simulink model "Grid_SensorLayout_SpatialAllignment_Clustering"  (R2018a)
settings: Solver=FixedStepAuto  StartTime=0.0  StopTime=SimulationTime  FixedStep=SamplingTime  RelTol=1e-3
values from neighbouring files (symbols this model uses):
  ValidateGRID = true    [SensorFusion_Script0_main.m]
  ValidateLAYOUT = true    [SensorFusion_Script0_main.m]
  VisualizeCLUSTERING = true    [SensorFusion_Script0_main.m]
undefined symbols (not defined in the file or in its folder): ACTIVATE_CAM, ACTIVATE_RAD, CAM1_detTimeStamp, CAM1_MeasNoise, CAM1_objClassID, CAM1_PX, CAM1_PY, CAM1_VX, CAM1_VY, CAM2_detTimeStamp, CAM2_MeasNoise, CAM2_objClassID, CAM2_PX, CAM2_PY, CAM2_VX, CAM2_VY, CAM3_detTimeStamp, CAM3_MeasNoise, CAM3_objClassID, CAM3_PX, CAM3_PY, CAM3_VX, CAM3_VY, CAM4_detTimeStamp, CAM4_MeasNoise, CAM4_objClassID, CAM4_PX, CAM4_PY, CAM4_VX, CAM4_VY, CAM5_detTimeStamp, CAM5_MeasNoise, CAM5_objClassID, CAM5_PX, CAM5_PY, CAM5_VX, CAM5_VY, CAM6_detTimeStamp, CAM6_MeasNoise, CAM6_objClassID, CAM6_PX, CAM6_PY, CAM6_VX, CAM6_VY, CAM7_detTimeStamp, CAM7_MeasNoise, CAM7_objClassID, CAM7_PX, CAM7_PY, CAM7_VX, CAM7_VY, CAM8_detTimeStamp, CAM8_MeasNoise, CAM8_objClassID, CAM8_PX, CAM8_PY, CAM8_VX, CAM8_VY, CAM_nMeas, CAM_TYPE ... (+171)
libraries: simulink_extras x4
(part 7 of 10)

== system Grid_SensorLayout_SpatialAllignment_Clustering/SENSOR_MEASUREMENTS/RADAR_CAMERA_EGO_SENSOR_INTERFACE/RoadSensors/LineSensor6/Subsystem1 ==
  CameraLineCoeff : Inport
  curv : Inport  Port=2
  curvRate : Inport  Port=3
  curvLen : Inport  Port=4
  alpha : Inport  Port=5
  ValidID : Inport  Port=6
  lateralOffset : Inport  Port=7
  xmin : Inport  Port=8
  xmax : Inport  Port=9
  lineWidth : Inport  Port=10
  TIME_STAMP : Inport  Port=11
  iter : Inport  Port=12
  Assignment : Assignment  DiagnosticForDimensions=Warning  IndexOptions=Index vector (port)  Indices=1  OutputSizes=1
  Bus Creator1 : BusCreator  Inputs=11  OutDataTypeStr=Bus: LineMeasParam  NonVirtualBus=on
  Bus Creator2 : BusCreator  Inputs=11  OutDataTypeStr=Bus: LineMeasParam  NonVirtualBus=on
  Constant1 : Constant  Value=single(10)
  Constant14 : Constant  Value=uint8(6)
  Constant2 : Constant  Value=single(10)
  Constant{35..39,43} (6 alike) : Constant  Value=single(0)
  Constant44 : Constant  Value=single(10)
  Switch : Switch  Criteria=u2 ~= 0
  C1 : Outport
  wires:
  Bus Creator1/1 -> Switch/3
  ValidID/1 -> Bus Creator1/2, Switch/2, Bus Creator2/2  "lineID"
  Bus Creator2/1 -> Switch/1
  CameraLineCoeff/1 -> Assignment/1
  Switch/1 -> Assignment/2
  iter/1 -> Assignment/3
  Assignment/1 -> C1/1
  TIME_STAMP/1 -> Bus Creator2/1  "TimeStamp"
  curv/1 -> Bus Creator2/4  "curvature"
  curvRate/1 -> Bus Creator2/5  "curvatureRate"
  curvLen/1 -> Bus Creator2/6  "curveLength"
  alpha/1 -> Bus Creator2/7  "HeadingAngle"
  lateralOffset/1 -> Bus Creator2/8  "LateralOffset"
  lineWidth/1 -> Bus Creator2/11  "LineMarkWidth"
  xmax/1 -> Bus Creator2/10  "validMinLongCoordLine"
  xmin/1 -> Bus Creator2/9  "validMaxLongCoordLine"
  Constant35/1 -> Bus Creator1/1  "TimeStamp"
  Constant14/1 -> Bus Creator2/3, Bus Creator1/3  "cameraID"
  Constant36/1 -> Bus Creator1/4  "curvature"
  Constant37/1 -> Bus Creator1/5  "curvatureRate"
  Constant38/1 -> Bus Creator1/6  "curveLength"
  Constant39/1 -> Bus Creator1/7  "HeadingAngle"
  Constant43/1 -> Bus Creator1/8  "LateralOffset"
  Constant44/1 -> Bus Creator1/9  "validMaxLongCoordLine"
  Constant1/1 -> Bus Creator1/10  "validMinLongCoordLine"
  Constant2/1 -> Bus Creator1/11  "LineMarkWidth"

== system Grid_SensorLayout_SpatialAllignment_Clustering/SENSOR_MEASUREMENTS/RADAR_CAMERA_EGO_SENSOR_INTERFACE/RoadSensors/LineSensor7/ExtractMeasParam1 ==
  idx : Inport
  time : Inport  Port=2
  Constant : Constant  Value=LINE_CURVATURE_CAM7
  Constant1 : Constant  Value=LINE_CURVDERIVATIVE_CAM7
  Constant2 : Constant  Value=LINE_CURVELENGTH_CAM7
  Constant3 : Constant  Value=LINE_HEADINGANGLE_CAM7
  Constant4 : Constant  Value=LINE_LATERALOFFSET_CAM7
  Constant5 : Constant  Value=LINE_XMIN_CAM7
  Constant6 : Constant  Value=LINE_detTimeStamp_CAM7
  Constant7 : Constant  Value=LINE_XMAX_CAM7
  Constant8 : Constant  Value=LINE_WIDTH_CAM7
  CurvLength : Selector  NumberOfDimensions=2  InputPortWidth=3  IndexOptions=Index vector (port),Index vector (port)  Indices=[1 3],1  OutputSizes=1,1
  Curvature : Selector  NumberOfDimensions=2  InputPortWidth=3  IndexOptions=Index vector (port),Index vector (port)  Indices=[1 3],1  OutputSizes=1,1
  CurvatureRate : Selector  NumberOfDimensions=2  InputPortWidth=3  IndexOptions=Index vector (port),Index vector (port)  Indices=[1 3],1  OutputSizes=1,1
  HeadingAngle : Selector  NumberOfDimensions=2  InputPortWidth=3  IndexOptions=Index vector (port),Index vector (port)  Indices=[1 3],1  OutputSizes=1,1
  LateralOffset : Selector  NumberOfDimensions=2  InputPortWidth=3  IndexOptions=Index vector (port),Index vector (port)  Indices=[1 3],1  OutputSizes=1,1
  lineWidth : Selector  NumberOfDimensions=2  InputPortWidth=3  IndexOptions=Index vector (port),Index vector (port)  Indices=[1 3],1  OutputSizes=1,1
  minValidX : Selector  NumberOfDimensions=2  InputPortWidth=3  IndexOptions=Index vector (port),Index vector (port)  Indices=[1 3],1  OutputSizes=1,1
  minValidY : Selector  NumberOfDimensions=2  InputPortWidth=3  IndexOptions=Index vector (port),Index vector (port)  Indices=[1 3],1  OutputSizes=1,1
  timeStamp : Selector  NumberOfDimensions=2  InputPortWidth=3  IndexOptions=Select all,Index vector (port)  Indices=[1 3],1  OutputSizes=1,1
  curvature : Outport
  curvRate : Outport  Port=2
  curvLength : Outport  Port=3
  headingAngle : Outport  Port=4
  lateralOffset : Outport  Port=5
  xmin : Outport  Port=6
  xmax : Outport  Port=7
  lineMarkWidth : Outport  Port=8
  measCaptureTime : Outport  Port=9
  wires:
  Constant3/1 -> HeadingAngle/1
  Constant2/1 -> CurvLength/1
  HeadingAngle/1 -> headingAngle/1
  Constant/1 -> Curvature/1
  Constant1/1 -> CurvatureRate/1
  CurvLength/1 -> curvLength/1
  Curvature/1 -> curvature/1
  CurvatureRate/1 -> curvRate/1
  Constant4/1 -> LateralOffset/1
  Constant5/1 -> minValidX/1
  Constant6/1 -> timeStamp/1
  timeStamp/1 -> measCaptureTime/1
  minValidX/1 -> xmin/1
  LateralOffset/1 -> lateralOffset/1
  minValidY/1 -> xmax/1
  Constant7/1 -> minValidY/1
  lineWidth/1 -> lineMarkWidth/1
  time/1 -> minValidX/2, minValidY/2, lineWidth/2, timeStamp/2, LateralOffset/2, HeadingAngle/2, CurvLength/2, CurvatureRate/2, Curvature/2
  idx/1 -> minValidX/3, lineWidth/3, minValidY/3, LateralOffset/3, HeadingAngle/3, CurvLength/3, CurvatureRate/3, Curvature/3
  Constant8/1 -> lineWidth/1

== system Grid_SensorLayout_SpatialAllignment_Clustering/SENSOR_MEASUREMENTS/RADAR_CAMERA_EGO_SENSOR_INTERFACE/RoadSensors/LineSensor7/IsValid2 ==
  LineID : Inport
  curvature : Inport  Port=2
  curvatureRate : Inport  Port=3
  curvLength : Inport  Port=4
  HeadingAngle : Inport  Port=5
  Abs{,1..3} (4 alike) : Abs
  Add : Sum  Inputs=++++
  Constant : Constant  Value=uint16(0)
  Data Type Conversion : DataTypeConversion  OutDataTypeStr=uint16
  Switch : Switch  Threshold=0.000001
  validID : Outport
  wires:
  Add/1 -> Switch/2
  Abs2/1 -> Add/3
  Constant/1 -> Switch/3
  Abs/1 -> Add/1
  curvature/1 -> Abs/1
  Abs3/1 -> Add/4
  Abs1/1 -> Add/2
  HeadingAngle/1 -> Abs3/1
  curvatureRate/1 -> Abs1/1
  curvLength/1 -> Abs2/1
  LineID/1 -> Data Type Conversion/1
  Switch/1 -> validID/1
  Data Type Conversion/1 -> Switch/1

== system Grid_SensorLayout_SpatialAllignment_Clustering/SENSOR_MEASUREMENTS/RADAR_CAMERA_EGO_SENSOR_INTERFACE/RoadSensors/LineSensor7/Subsystem1 ==
  CameraLineCoeff : Inport
  curv : Inport  Port=2
  curvRate : Inport  Port=3
  curvLen : Inport  Port=4
  alpha : Inport  Port=5
  ValidID : Inport  Port=6
  lateralOffset : Inport  Port=7
  xmin : Inport  Port=8
  xmax : Inport  Port=9
  lineWidth : Inport  Port=10
  TIME_STAMP : Inport  Port=11
  iter : Inport  Port=12
  Assignment : Assignment  DiagnosticForDimensions=Warning  IndexOptions=Index vector (port)  Indices=1  OutputSizes=1
  Bus Creator1 : BusCreator  Inputs=11  OutDataTypeStr=Bus: LineMeasParam  NonVirtualBus=on
  Bus Creator2 : BusCreator  Inputs=11  OutDataTypeStr=Bus: LineMeasParam  NonVirtualBus=on
  Constant1 : Constant  Value=single(10)
  Constant14 : Constant  Value=uint8(7)
  Constant2 : Constant  Value=single(10)
  Constant{35..39,43} (6 alike) : Constant  Value=single(0)
  Constant44 : Constant  Value=single(10)
  Switch : Switch  Criteria=u2 ~= 0
  C1 : Outport
  wires:
  Bus Creator1/1 -> Switch/3
  ValidID/1 -> Bus Creator1/2, Switch/2, Bus Creator2/2  "lineID"
  Bus Creator2/1 -> Switch/1
  CameraLineCoeff/1 -> Assignment/1
  Switch/1 -> Assignment/2
  iter/1 -> Assignment/3
  Assignment/1 -> C1/1
  TIME_STAMP/1 -> Bus Creator2/1  "TimeStamp"
  curv/1 -> Bus Creator2/4  "curvature"
  curvRate/1 -> Bus Creator2/5  "curvatureRate"
  curvLen/1 -> Bus Creator2/6  "curveLength"
  alpha/1 -> Bus Creator2/7  "HeadingAngle"
  lateralOffset/1 -> Bus Creator2/8  "LateralOffset"
  lineWidth/1 -> Bus Creator2/11  "LineMarkWidth"
  xmax/1 -> Bus Creator2/10  "validMinLongCoordLine"
  xmin/1 -> Bus Creator2/9  "validMaxLongCoordLine"
  Constant35/1 -> Bus Creator1/1  "TimeStamp"
  Constant14/1 -> Bus Creator2/3, Bus Creator1/3  "cameraID"
  Constant36/1 -> Bus Creator1/4  "curvature"
  Constant37/1 -> Bus Creator1/5  "curvatureRate"
  Constant38/1 -> Bus Creator1/6  "curveLength"
  Constant39/1 -> Bus Creator1/7  "HeadingAngle"
  Constant43/1 -> Bus Creator1/8  "LateralOffset"
  Constant44/1 -> Bus Creator1/9  "validMaxLongCoordLine"
  Constant1/1 -> Bus Creator1/10  "validMinLongCoordLine"
  Constant2/1 -> Bus Creator1/11  "LineMarkWidth"

== system Grid_SensorLayout_SpatialAllignment_Clustering/SENSOR_MEASUREMENTS/RADAR_CAMERA_EGO_SENSOR_INTERFACE/RoadSensors/LineSensor8/ExtractMeasParam1 ==
  idx : Inport
  time : Inport  Port=2
  Constant : Constant  Value=LINE_CURVATURE_CAM8
  Constant1 : Constant  Value=LINE_CURVDERIVATIVE_CAM8
  Constant2 : Constant  Value=LINE_CURVELENGTH_CAM8
  Constant3 : Constant  Value=LINE_HEADINGANGLE_CAM8
  Constant4 : Constant  Value=LINE_LATERALOFFSET_CAM8
  Constant5 : Constant  Value=LINE_XMIN_CAM8
  Constant6 : Constant  Value=LINE_detTimeStamp_CAM8
  Constant7 : Constant  Value=LINE_XMAX_CAM8
  Constant8 : Constant  Value=LINE_WIDTH_CAM8
  CurvLength : Selector  NumberOfDimensions=2  InputPortWidth=3  IndexOptions=Index vector (port),Index vector (port)  Indices=[1 3],1  OutputSizes=1,1
  Curvature : Selector  NumberOfDimensions=2  InputPortWidth=3  IndexOptions=Index vector (port),Index vector (port)  Indices=[1 3],1  OutputSizes=1,1
  CurvatureRate : Selector  NumberOfDimensions=2  InputPortWidth=3  IndexOptions=Index vector (port),Index vector (port)  Indices=[1 3],1  OutputSizes=1,1
  HeadingAngle : Selector  NumberOfDimensions=2  InputPortWidth=3  IndexOptions=Index vector (port),Index vector (port)  Indices=[1 3],1  OutputSizes=1,1
  LateralOffset : Selector  NumberOfDimensions=2  InputPortWidth=3  IndexOptions=Index vector (port),Index vector (port)  Indices=[1 3],1  OutputSizes=1,1
  lineWidth : Selector  NumberOfDimensions=2  InputPortWidth=3  IndexOptions=Index vector (port),Index vector (port)  Indices=[1 3],1  OutputSizes=1,1
  minValidX : Selector  NumberOfDimensions=2  InputPortWidth=3  IndexOptions=Index vector (port),Index vector (port)  Indices=[1 3],1  OutputSizes=1,1
  minValidY : Selector  NumberOfDimensions=2  InputPortWidth=3  IndexOptions=Index vector (port),Index vector (port)  Indices=[1 3],1  OutputSizes=1,1
  timeStamp : Selector  NumberOfDimensions=2  InputPortWidth=3  IndexOptions=Select all,Index vector (port)  Indices=[1 3],1  OutputSizes=1,1
  curvature : Outport
  curvRate : Outport  Port=2
  curvLength : Outport  Port=3
  headingAngle : Outport  Port=4
  lateralOffset : Outport  Port=5
  xmin : Outport  Port=6
  xmax : Outport  Port=7
  lineMarkWidth : Outport  Port=8
  measCaptureTime : Outport  Port=9
  wires:
  Constant3/1 -> HeadingAngle/1
  Constant2/1 -> CurvLength/1
  HeadingAngle/1 -> headingAngle/1
  Constant/1 -> Curvature/1
  Constant1/1 -> CurvatureRate/1
  CurvLength/1 -> curvLength/1
  Curvature/1 -> curvature/1
  CurvatureRate/1 -> curvRate/1
  Constant4/1 -> LateralOffset/1
  Constant5/1 -> minValidX/1
  Constant6/1 -> timeStamp/1
  timeStamp/1 -> measCaptureTime/1
  minValidX/1 -> xmin/1
  LateralOffset/1 -> lateralOffset/1
  minValidY/1 -> xmax/1
  Constant7/1 -> minValidY/1
  lineWidth/1 -> lineMarkWidth/1
  time/1 -> minValidX/2, minValidY/2, lineWidth/2, timeStamp/2, LateralOffset/2, HeadingAngle/2, CurvLength/2, CurvatureRate/2, Curvature/2
  idx/1 -> minValidX/3, lineWidth/3, minValidY/3, LateralOffset/3, HeadingAngle/3, CurvLength/3, CurvatureRate/3, Curvature/3
  Constant8/1 -> lineWidth/1

== system Grid_SensorLayout_SpatialAllignment_Clustering/SENSOR_MEASUREMENTS/RADAR_CAMERA_EGO_SENSOR_INTERFACE/RoadSensors/LineSensor8/IsValid2 ==
  LineID : Inport
  curvature : Inport  Port=2
  curvatureRate : Inport  Port=3
  curvLength : Inport  Port=4
  HeadingAngle : Inport  Port=5
  Abs{,1..3} (4 alike) : Abs
  Add : Sum  Inputs=++++
  Constant : Constant  Value=uint16(0)
  Data Type Conversion : DataTypeConversion  OutDataTypeStr=uint16
  Switch : Switch  Threshold=0.000001
  validID : Outport
  wires:
  Add/1 -> Switch/2
  Abs2/1 -> Add/3
  Constant/1 -> Switch/3
  Abs/1 -> Add/1
  curvature/1 -> Abs/1
  Abs3/1 -> Add/4
  Abs1/1 -> Add/2
  HeadingAngle/1 -> Abs3/1
  curvatureRate/1 -> Abs1/1
  curvLength/1 -> Abs2/1
  LineID/1 -> Data Type Conversion/1
  Switch/1 -> validID/1
  Data Type Conversion/1 -> Switch/1

== system Grid_SensorLayout_SpatialAllignment_Clustering/SENSOR_MEASUREMENTS/RADAR_CAMERA_EGO_SENSOR_INTERFACE/RoadSensors/LineSensor8/Subsystem1 ==
  CameraLineCoeff : Inport
  curv : Inport  Port=2
  curvRate : Inport  Port=3
  curvLen : Inport  Port=4
  alpha : Inport  Port=5
  ValidID : Inport  Port=6
  lateralOffset : Inport  Port=7
  xmin : Inport  Port=8
  xmax : Inport  Port=9
  lineWidth : Inport  Port=10
  TIME_STAMP : Inport  Port=11
  iter : Inport  Port=12
  Assignment : Assignment  DiagnosticForDimensions=Warning  IndexOptions=Index vector (port)  Indices=1  OutputSizes=1
  Bus Creator1 : BusCreator  Inputs=11  OutDataTypeStr=Bus: LineMeasParam  NonVirtualBus=on
  Bus Creator2 : BusCreator  Inputs=11  OutDataTypeStr=Bus: LineMeasParam  NonVirtualBus=on
  Constant1 : Constant  Value=single(10)
  Constant14 : Constant  Value=uint8(8)
  Constant2 : Constant  Value=single(10)
  Constant{35..39,43} (6 alike) : Constant  Value=single(0)
  Constant44 : Constant  Value=single(10)
  Switch : Switch  Criteria=u2 ~= 0
  C1 : Outport
  wires:
  Bus Creator1/1 -> Switch/3
  ValidID/1 -> Bus Creator1/2, Switch/2, Bus Creator2/2  "lineID"
  Bus Creator2/1 -> Switch/1
  CameraLineCoeff/1 -> Assignment/1
  Switch/1 -> Assignment/2
  iter/1 -> Assignment/3
  Assignment/1 -> C1/1
  TIME_STAMP/1 -> Bus Creator2/1  "TimeStamp"
  curv/1 -> Bus Creator2/4  "curvature"
  curvRate/1 -> Bus Creator2/5  "curvatureRate"
  curvLen/1 -> Bus Creator2/6  "curveLength"
  alpha/1 -> Bus Creator2/7  "HeadingAngle"
  lateralOffset/1 -> Bus Creator2/8  "LateralOffset"
  lineWidth/1 -> Bus Creator2/11  "LineMarkWidth"
  xmax/1 -> Bus Creator2/10  "validMinLongCoordLine"
  xmin/1 -> Bus Creator2/9  "validMaxLongCoordLine"
  Constant35/1 -> Bus Creator1/1  "TimeStamp"
  Constant14/1 -> Bus Creator2/3, Bus Creator1/3  "cameraID"
  Constant36/1 -> Bus Creator1/4  "curvature"
  Constant37/1 -> Bus Creator1/5  "curvatureRate"
  Constant38/1 -> Bus Creator1/6  "curveLength"
  Constant39/1 -> Bus Creator1/7  "HeadingAngle"
  Constant43/1 -> Bus Creator1/8  "LateralOffset"
  Constant44/1 -> Bus Creator1/9  "validMaxLongCoordLine"
  Constant1/1 -> Bus Creator1/10  "validMinLongCoordLine"
  Constant2/1 -> Bus Creator1/11  "LineMarkWidth"

== system Grid_SensorLayout_SpatialAllignment_Clustering/OBJECT_TRACKER_SENSOR_FUSION/NEAREST_NEIGHBOUR_FOR_CAMERA_MEASUREMENT_GROUPING/NN_MEASUREMENT_GROUPING_WITHIN_EPS/For Iterator Subsystem/NN/PERFORM_NN_CLUSTERING ==
  nMeas : Inport
  measArray : Inport  Port=2
  CLSTR_DATA : Inport  Port=3
  idx_i : Inport  Port=4
  CHECK_CONDITION : Subsystem
  For Iterator : ForIterator  ResetStates=reset  IterationSource=external
  SET_DATA : Subsystem
  CLSTR_DATA_UPD : Outport
  wires:
  nMeas/1 -> For Iterator/1
  idx_i/1 -> CHECK_CONDITION/2(idx_i)
  measArray/1 -> CHECK_CONDITION/1(MEAS)
  For Iterator/1 -> [y_j], CHECK_CONDITION/3(idx_j)
  CHECK_CONDITION/1(isMember) -> SET_DATA/1(isClusterMember)
  SET_DATA/1(CLSTR_DATA_UPD) -> CHECK_CONDITION/5(CLSTR_DATA_PREV), CLSTR_DATA_UPD/1
  CLSTR_DATA/1 -> CHECK_CONDITION/4(CLSTR_DATA_INIT)
  CHECK_CONDITION/2(CLSTR_DATA) -> SET_DATA/2(CLSTR_DATA)
  [y_j] -> SET_DATA/3(idx_j)

== system Grid_SensorLayout_SpatialAllignment_Clustering/OBJECT_TRACKER_SENSOR_FUSION/NEAREST_NEIGHBOUR_FOR_CAMERA_MEASUREMENT_GROUPING/NN_MEASUREMENT_GROUPING_WITHIN_EPS/For Iterator Subsystem/NN/SET_CLUSTER_ID_AND_UPDATE_NUMBER_OF_CLUSTERS ==
  CLUSTERING_DATA : Inport
  CAM_MEAS_CTS : Inport  Port=2
  Add2 : Sum
  Bus Creator : BusCreator  Inputs=7  OutDataTypeStr=Bus: CLUSTER_DATA_STRUCT_SNSR  NonVirtualBus=on
      settings: InheritFromInputs=off
  Bus Selector : BusSelector  OutputSignals=nClusters
  Bus Selector1 : BusSelector  OutputSignals=ValidCumulativeMeasCount
  Bus Selector2 : BusSelector  OutputSignals=ClusterCenter,ClusterCovariance,ClusterSizes,ClusterToMeasAssignment,isMeasVisitedFlag,nClusters,ClusterMember
  Constant3 : Constant  Value=uint16(1)
  Data Type Conversion : DataTypeConversion  OutDataTypeStr=uint16
  Selector : Selector  NumberOfDimensions=2  InputPortWidth=3  IndexOptions=Select all,Index vector (port)  Indices=[1 3],1  OutputSizes=1,1
  Terminator1 : Terminator
  Width : Width
  nRadMeas : Outport
  CLUSTER_DATA : Outport  Port=2
  wires:
  CLUSTERING_DATA/1 -> Bus Selector2/1, Bus Selector/1
  Bus Selector/1 -> Add2/1  "<nClusters>"
  CAM_MEAS_CTS/1 -> Bus Selector1/1
  Add2/1 -> Data Type Conversion/1
  Constant3/1 -> Add2/2
  Data Type Conversion/1 -> [B]
  Bus Selector2/1 -> Bus Creator/1  "<ClusterCenter>"
  Bus Selector2/2 -> Bus Creator/2  "<ClusterCovariance>"
  Bus Selector2/3 -> Bus Creator/3  "<ClusterSizes>"
  Bus Selector2/4 -> Bus Creator/4  "<ClusterToMeasAssignment>"
  Bus Selector2/5 -> Bus Creator/5  "<isMeasVisitedFlag>"
  Bus Selector2/7 -> Bus Creator/7  "<ClusterMember>"
  Bus Selector2/6 -> Terminator1/1  "<nClusters>"
  [B] -> Bus Creator/6  "nClusters"
  Bus Creator/1 -> CLUSTER_DATA/1
  Bus Selector1/1 -> Width/1, Selector/1  "<ValidCumulativeMeasCount>"
  Width/1 -> Selector/2
  Selector/1 -> nRadMeas/1

== system Grid_SensorLayout_SpatialAllignment_Clustering/OBJECT_TRACKER_SENSOR_FUSION/NEAREST_NEIGHBOUR_FOR_CAMERA_MEASUREMENT_GROUPING/NN_MEASUREMENT_GROUPING_WITHIN_EPS/For Iterator Subsystem/NN/Subsystem ==
  CLSTR_DATA : Inport
  Bus Selector : BusSelector  OutputSignals=ClusterSizes,nClusters
  Selector : Selector  NumberOfDimensions=2  InputPortWidth=3  IndexOptions=Select all,Index vector (port)  Indices=[1 3],1  OutputSizes=1,1
  ClstrSize : Outport
  wires:
  Bus Selector/2 -> Selector/2  "<nClusters>"
  Bus Selector/1 -> Selector/1  "<ClusterSizes>"
  CLSTR_DATA/1 -> Bus Selector/1
  Selector/1 -> ClstrSize/1

== system Grid_SensorLayout_SpatialAllignment_Clustering/OBJECT_TRACKER_SENSOR_FUSION/SENSOR_LAYOUT_AND_CHRACTERIZATION/PRE_COMPUTE_SENSOR_FOV_GRID/COMPUTE_CAMERA_SNSR_GRID/ComputeCoverageANDConfidence/Compute_Cell_X_and_Y_index ==
  CellIndex : Inport
  GridID_vec : Inport  Port=2
  GridParam : Inport  Port=3
  SensorExtrinsicParam : Inport  Port=4
  SensorIntrinsicParam : Inport  Port=5
  Compute_Cell_X_Y_Center_Coordinate : Subsystem
  Compute_FOV_Overlap_with_Cell_and_Region_Confidence : Subsystem
  GET_DATA : Subsystem
  Transform_Cell_Coordinate_Vehicle_Frame_To_Sensor_Frame : Subsystem
  RegionConfidence : Outport
  FOVOverlap : Outport  Port=2
  wires:
  GridID_vec/1 -> GET_DATA/1(GridID_vector)
  CellIndex/1 -> GET_DATA/2(index)
  GridParam/1 -> GET_DATA/3(GridParam)
  GET_DATA/1(CellID) -> Compute_Cell_X_Y_Center_Coordinate/1(Cell_id)
  GET_DATA/2(<xRes>) -> Compute_Cell_X_Y_Center_Coordinate/2(xRes)
  GET_DATA/3(<xRear>) -> Compute_Cell_X_Y_Center_Coordinate/3(xRear)
  GET_DATA/4(<nGridCellsLat>) -> Compute_Cell_X_Y_Center_Coordinate/4(Cy)
  GET_DATA/5(<yRes>) -> Compute_Cell_X_Y_Center_Coordinate/5(yRes)
  GET_DATA/6(<yLeft>) -> Compute_Cell_X_Y_Center_Coordinate/6(yLeft)
  SensorExtrinsicParam/1 -> Transform_Cell_Coordinate_Vehicle_Frame_To_Sensor_Frame/3(SensorExtrinsic)
  Compute_Cell_X_Y_Center_Coordinate/1(CellCenterCoordX) -> Transform_Cell_Coordinate_Vehicle_Frame_To_Sensor_Frame/1(Cell_xCoord)
  Compute_Cell_X_Y_Center_Coordinate/2(CellCenterCoordY) -> Transform_Cell_Coordinate_Vehicle_Frame_To_Sensor_Frame/2(Cell_y_Coord)
  Transform_Cell_Coordinate_Vehicle_Frame_To_Sensor_Frame/1(Cell_xSnsrCoord) -> Compute_FOV_Overlap_with_Cell_and_Region_Confidence/1(Cell_xSnsrCoord)
  Transform_Cell_Coordinate_Vehicle_Frame_To_Sensor_Frame/2(Cell_ySnsrCoord) -> Compute_FOV_Overlap_with_Cell_and_Region_Confidence/2(Cell_ySnsrCoord)
  SensorIntrinsicParam/1 -> Compute_FOV_Overlap_with_Cell_and_Region_Confidence/3(SnsrIntrinsic)
  Compute_FOV_Overlap_with_Cell_and_Region_Confidence/1(RegionConfidence) -> RegionConfidence/1
  Compute_FOV_Overlap_with_Cell_and_Region_Confidence/2(FOVOverlap) -> FOVOverlap/1

== system Grid_SensorLayout_SpatialAllignment_Clustering/OBJECT_TRACKER_SENSOR_FUSION/SENSOR_LAYOUT_AND_CHRACTERIZATION/PRE_COMPUTE_SENSOR_FOV_GRID/COMPUTE_CAMERA_SNSR_GRID/ComputeCoverageANDConfidence/SET_DATA ==
  GridIndex : Inport
  RegionConfiArray : Inport  Port=2
  FOVOverlapArray : Inport  Port=3
  SnsrIndex : Inport  Port=4
  confi : Inport  Port=5
  overlap : Inport  Port=6
  Assignment : Assignment  NumberOfDimensions=2  DiagnosticForDimensions=Warning  IndexOptions=Index vector (port),Index vector (port)  Indices=1,1  OutputSizes=1,1
  Assignment1 : Assignment  NumberOfDimensions=2  DiagnosticForDimensions=Warning  IndexOptions=Index vector (port),Index vector (port)  Indices=1,1  OutputSizes=1,1
  RegionConfidence : Outport
  FOVOverlap : Outport  Port=2
  wires:
  SnsrIndex/1 -> Assignment1/3, Assignment/3
  RegionConfiArray/1 -> Assignment/1
  Assignment/1 -> RegionConfidence/1
  GridIndex/1 -> Assignment/4, Assignment1/4
  Assignment1/1 -> FOVOverlap/1
  overlap/1 -> Assignment1/2
  FOVOverlapArray/1 -> Assignment1/1
  confi/1 -> Assignment/2

== system Grid_SensorLayout_SpatialAllignment_Clustering/OBJECT_TRACKER_SENSOR_FUSION/SENSOR_LAYOUT_AND_CHRACTERIZATION/PRE_COMPUTE_SENSOR_FOV_GRID/COMPUTE_RADAR_SNSR_GRID/ComputeCoverageANDConfidence/Compute_Cell_X_and_Y_index ==
  CellIndex : Inport
  GridID_vec : Inport  Port=2
  GridParam : Inport  Port=3
  SensorExtrinsicParam : Inport  Port=4
  SensorIntrinsicParam : Inport  Port=5
  Compute_Cell_X_Y_Center_Coordinate : Subsystem
  Compute_FOV_Overlap_with_Cell_and_Region_Confidence : Subsystem
  GET_DATA : Subsystem
  Transform_Cell_Coordinate_Vehicle_Frame_To_Sensor_Frame : Subsystem
  RegionConfidence : Outport
  FOVOverlap : Outport  Port=2
  wires:
  GridID_vec/1 -> GET_DATA/1(GridID_vector)
  CellIndex/1 -> GET_DATA/2(index)
  GridParam/1 -> GET_DATA/3(GridParam)
  GET_DATA/1(CellID) -> Compute_Cell_X_Y_Center_Coordinate/1(Cell_id)
  GET_DATA/2(<xRes>) -> Compute_Cell_X_Y_Center_Coordinate/2(xRes)
  GET_DATA/3(<xRear>) -> Compute_Cell_X_Y_Center_Coordinate/3(xRear)
  GET_DATA/4(<nGridCellsLat>) -> Compute_Cell_X_Y_Center_Coordinate/4(Cy)
  GET_DATA/5(<yRes>) -> Compute_Cell_X_Y_Center_Coordinate/5(yRes)
  GET_DATA/6(<yLeft>) -> Compute_Cell_X_Y_Center_Coordinate/6(yLeft)
  SensorExtrinsicParam/1 -> Transform_Cell_Coordinate_Vehicle_Frame_To_Sensor_Frame/3(SensorExtrinsic)
  Compute_Cell_X_Y_Center_Coordinate/1(CellCenterCoordX) -> Transform_Cell_Coordinate_Vehicle_Frame_To_Sensor_Frame/1(Cell_xCoord)
  Compute_Cell_X_Y_Center_Coordinate/2(CellCenterCoordY) -> Transform_Cell_Coordinate_Vehicle_Frame_To_Sensor_Frame/2(Cell_y_Coord)
  Transform_Cell_Coordinate_Vehicle_Frame_To_Sensor_Frame/1(Cell_xSnsrCoord) -> Compute_FOV_Overlap_with_Cell_and_Region_Confidence/1(Cell_xSnsrCoord)
  Transform_Cell_Coordinate_Vehicle_Frame_To_Sensor_Frame/2(Cell_ySnsrCoord) -> Compute_FOV_Overlap_with_Cell_and_Region_Confidence/2(Cell_ySnsrCoord)
  SensorIntrinsicParam/1 -> Compute_FOV_Overlap_with_Cell_and_Region_Confidence/3(SnsrIntrinsic)
  Compute_FOV_Overlap_with_Cell_and_Region_Confidence/1(RegionConfidence) -> RegionConfidence/1
  Compute_FOV_Overlap_with_Cell_and_Region_Confidence/2(FOVOverlap) -> FOVOverlap/1

== system Grid_SensorLayout_SpatialAllignment_Clustering/OBJECT_TRACKER_SENSOR_FUSION/SENSOR_LAYOUT_AND_CHRACTERIZATION/PRE_COMPUTE_SENSOR_FOV_GRID/COMPUTE_RADAR_SNSR_GRID/ComputeCoverageANDConfidence/SET_DATA ==
  GridIndex : Inport
  RegionConfiArray : Inport  Port=2
  FOVOverlapArray : Inport  Port=3
  SnsrIndex : Inport  Port=4
  confi : Inport  Port=5
  overlap : Inport  Port=6
  Assignment : Assignment  NumberOfDimensions=2  DiagnosticForDimensions=Warning  IndexOptions=Index vector (port),Index vector (port)  Indices=1,1  OutputSizes=1,1
  Assignment1 : Assignment  NumberOfDimensions=2  DiagnosticForDimensions=Warning  IndexOptions=Index vector (port),Index vector (port)  Indices=1,1  OutputSizes=1,1
  RegionConfidence : Outport
  FOVOverlap : Outport  Port=2
  wires:
  SnsrIndex/1 -> Assignment1/3, Assignment/3
  RegionConfiArray/1 -> Assignment/1
  Assignment/1 -> RegionConfidence/1
  GridIndex/1 -> Assignment/4, Assignment1/4
  Assignment1/1 -> FOVOverlap/1
  overlap/1 -> Assignment1/2
  FOVOverlapArray/1 -> Assignment1/1
  confi/1 -> Assignment/2

== system Grid_SensorLayout_SpatialAllignment_Clustering/OBJECT_TRACKER_SENSOR_FUSION/SENSOR_LAYOUT_AND_CHRACTERIZATION/PRE_COMPUTE_SENSOR_FOV_GRID/CREATE_GRID/For Iterator Subsystem/Compute_Grid_Cell_Cartesian_Coordinate ==
  note: Get_Grid_Limits_Data
  note: Compute_Grid_Cell_x_Coordinate
  note: Compute_Grid_Cell_y_Coordinate
  GridParam : Inport
  x_Index : Inport  Port=2
  y_Index : Inport  Port=3
  Add : Sum
  Add1 : Sum
  Bus Selector : BusSelector  OutputSignals=xRes,xRear
  Bus Selector1 : BusSelector  OutputSignals=yRes,yLeft
  Bus Selector2 : BusSelector  OutputSignals=xGridParameters,yGridParameters
  Constant : Constant  Value=single(1)
  Multiply : Product
  Multiply1 : Product
  Subtract : Sum  Inputs=+-
  Subtract1 : Sum  Inputs=-+
  x_Coordinate : Outport
  y_Coordinate : Outport  Port=2
  wires:
  [xRes] -> Multiply/2
  Add/1 -> x_Coordinate/1
  Subtract/1 -> Multiply/1
  Constant/1 -> Subtract/2, Subtract1/1
  [xRear] -> Add/2
  Multiply/1 -> Add/1
  [yRes] -> Multiply1/2
  y_Index/1 -> Subtract1/2
  Add1/1 -> y_Coordinate/1
  Multiply1/1 -> Add1/1
  Subtract1/1 -> Multiply1/1
  [yLeft] -> Add1/2
  Bus Selector/1 -> [xRes]  "<xRes>"
  Bus Selector1/1 -> [yRes]  "<yRes>"
  Bus Selector1/2 -> [yLeft]  "<yLeft>"
  Bus Selector/2 -> [xRear]  "<xRear>"
  x_Index/1 -> Subtract/1
  Bus Selector2/1 -> Bus Selector/1  "<xGridParameters>"
  GridParam/1 -> Bus Selector2/1
  Bus Selector2/2 -> Bus Selector1/1  "<yGridParameters>"

== system Grid_SensorLayout_SpatialAllignment_Clustering/OBJECT_TRACKER_SENSOR_FUSION/SENSOR_LAYOUT_AND_CHRACTERIZATION/PRE_COMPUTE_SENSOR_FOV_GRID/CREATE_GRID/For Iterator Subsystem/Compute_Grid_Cell_Discreete_Index ==
  note: Get_Data
  note: 2D_Cell_Index_To_1D_Cell_Index
  note: Compute_Grid_X_Index
  note: Compute_x_index
  note: Compute_x_index_Lower_Limit
  note: Translate_x_index_to_make_it_positive
  note: Compute_Grid_Y_Index
  note: Compute_y_index
  note: Translate_y_index_to_make_it_positive
  note: Compute_y_index_Lower_Limit
  GridParam : Inport
  x_coord : Inport  Port=2
  y_coord : Inport  Port=3
  Add : Sum
  Bus Selector : BusSelector  OutputSignals=xRes,xRear
  Bus Selector1 : BusSelector  OutputSignals=nGridCellsLat,yRes,yLeft
  Bus Selector2 : BusSelector  OutputSignals=xGridParameters,yGridParameters
  Divide : Product  Inputs=*/
  Divide1 : Product  Inputs=*/
  Divide2 : Product  Inputs=/*
  Divide3 : Product  Inputs=/*
  Floor{,1..3} (4 alike) : Rounding
  Minus : Sum  Inputs=+-
  Minus1 : Sum  Inputs=+-
  Multiply : Product
  CellID_x : Outport
  CellID_y : Outport  Port=2
  CellID : Outport  Port=3
  wires:
  Minus/1 -> Multiply/1, CellID_x/1
  Floor/1 -> Minus/1
  Floor2/1 -> Minus/2
  Divide/1 -> Floor/1
  Divide2/1 -> Floor2/1
  x_coord/1 -> Divide/1
  [xRes] -> Divide2/1, Divide/2
  [xRear] -> Divide2/2
  y_coord/1 -> Divide1/1
  [yRes] -> Divide3/1, Divide1/2
  [yLeft] -> Divide3/2
  Floor3/1 -> Minus1/2
  Divide3/1 -> Floor3/1
  Divide1/1 -> Floor1/1
  Floor1/1 -> Minus1/1
  Minus1/1 -> Add/2, CellID_y/1
  [Cy] -> Multiply/2
  Multiply/1 -> Add/1
  Add/1 -> CellID/1
  Bus Selector/2 -> [xRear]  "<xRear>"
  Bus Selector2/1 -> Bus Selector/1  "<xGridParameters>"
  GridParam/1 -> Bus Selector2/1
  Bus Selector2/2 -> Bus Selector1/1  "<yGridParameters>"
  Bus Selector/1 -> [xRes]  "<xRes>"
  Bus Selector1/3 -> [yLeft]  "<yLeft>"
  Bus Selector1/2 -> [yRes]  "<yRes>"
  Bus Selector1/1 -> [Cy]  "<nGridCellsLat>"

== system Grid_SensorLayout_SpatialAllignment_Clustering/OBJECT_TRACKER_SENSOR_FUSION/SENSOR_LAYOUT_AND_CHRACTERIZATION/PRE_COMPUTE_SENSOR_FOV_GRID/CREATE_GRID/For Iterator Subsystem/SET_DATA ==
  CellIDArray : Inport
  CellID : Inport  Port=2
  Assignment : Assignment  NumberOfDimensions=2  DiagnosticForDimensions=Warning  IndexOptions=Assign all,Index vector (port)  Indices=1,1  OutputSizes=1,1
  Constant2 : Constant  Value=int32(1)
  Data Type Conversion1 : DataTypeConversion  OutDataTypeStr=int32
  Data Type Conversion3 : DataTypeConversion  OutDataTypeStr=int32
  Reshape : Reshape  OutputDimensionality=Row vector (2-D)
  Subtract : Sum
  CellIDArrayUpd : Outport
  wires:
  CellIDArray/1 -> Reshape/1
  Assignment/1 -> CellIDArrayUpd/1
  Constant2/1 -> Subtract/2
  CellID/1 -> Data Type Conversion1/1, Assignment/2
  Data Type Conversion3/1 -> Assignment/3
  Data Type Conversion1/1 -> Subtract/1
  Subtract/1 -> Data Type Conversion3/1
  Reshape/1 -> Assignment/1

== system Grid_SensorLayout_SpatialAllignment_Clustering/OBJECT_TRACKER_SENSOR_FUSION/SENSOR_LAYOUT_AND_CHRACTERIZATION/SET_SENSOR_CALLIBRATION_PARAMETER/SET_CAMERA_SENSOR_PARAM/SET_CAMERA_EXTRINSIC_PARAM/SET_CAMERA_EXTRINSIC_PARAM ==
  SensorParam : Inport
  SensorID : Inport  Port=2
  Assignment : Assignment  DiagnosticForDimensions=Warning  IndexOptions=Index vector (port)  Indices=1  OutputSizes=1
  Bus Creator : BusCreator  Inputs=12  OutDataTypeStr=Bus: CameraExtrinsicParam  NonVirtualBus=on
  Bus Selector : BusSelector  OutputSignals=CameraID,CameraType,isActive,RotMat2D,TranslationVec,MountX,MountY,MountZ,MountYaw,MountPitch,MountRoll,nMeas
  Constant : Constant  Value=ACTIVATE_CAM
  Constant1 : Constant  Value=CAM_X_INSTALL
  Constant2 : Constant  Value=CAM_Y_INSTALL
  Constant3 : Constant  Value=CAM_YAW_INSTALL
  Constant4 : Constant  Value=CAM_nMeas
  Constant9 : Constant  Value=CAM_TYPE
  CreateRotationMatTranslationVector : Subsystem
  Data Type Conversion : DataTypeConversion  OutDataTypeStr=uint8
  Selector{,1..5,8} (7 alike) : Selector  InputPortWidth=nCameras  IndexOptions=Index vector (port)  Indices=[1 3]  OutputSizes=1
  Terminator{,1..8} (9 alike) : Terminator
  Out1 : Outport
  wires:
  Assignment/1 -> Out1/1
  Constant/1 -> Selector1/1
  SensorParam/1 -> [Param], Selector/1
  Constant2/1 -> Selector3/1
  [SensorID] -> Selector5/2, Selector4/2, Selector3/2, Selector2/2, Selector1/2, Selector8/2, Data Type Conversion/1
  Constant3/1 -> Selector4/1
  Constant1/1 -> Selector2/1
  Selector/1 -> Bus Selector/1
  Bus Creator/1 -> Assignment/2
  Bus Selector/1 -> Terminator/1  "<CameraID>"
  SensorID/1 -> [SensorID], Selector/2
  [Param] -> Assignment/1
  [SensorID] -> Assignment/3
  Selector2/1 -> [MountX], Bus Creator/6  "MountX"
  Selector3/1 -> [MountY], Bus Creator/7  "MountY"
  [MountX] -> CreateRotationMatTranslationVector/2(xMount)
  [MountY] -> CreateRotationMatTranslationVector/3(yMount)
  Selector4/1 -> [MountYaw], Bus Creator/9  "MountYaw"
  [MountYaw] -> CreateRotationMatTranslationVector/1(yawInstall)
  CreateRotationMatTranslationVector/1(RotMatrx) -> [RotMat]
  CreateRotationMatTranslationVector/2(TranslationVector) -> [TransVec]
  Data Type Conversion/1 -> Bus Creator/1  "CameraID"
  Selector8/1 -> Bus Creator/2  "CameraType"
  Constant9/1 -> Selector8/1
  Selector1/1 -> Bus Creator/3  "isActive"
  [RotMat] -> Bus Creator/4  "RotMat2D"
  [TransVec] -> Bus Creator/5  "TranslationVec"
  Bus Selector/2 -> Terminator1/1  "<CameraType>"
  Bus Selector/3 -> Terminator2/1  "<isActive>"
  Bus Selector/4 -> Terminator3/1  "<RotMat2D>"
  Bus Selector/8 -> Bus Creator/8  "<MountZ>"
  Bus Selector/5 -> Terminator4/1  "<TranslationVec>"
  Bus Selector/7 -> Terminator6/1  "<MountY>"
  Bus Selector/6 -> Terminator5/1  "<MountX>"
  Bus Selector/9 -> Terminator8/1  "<MountYaw>"
  Bus Selector/11 -> Bus Creator/11  "<MountRoll>"
  Bus Selector/10 -> Bus Creator/10  "<MountPitch>"
  Selector5/1 -> Bus Creator/12  "nMeas"
  Constant4/1 -> Selector5/1
  Bus Selector/12 -> Terminator7/1  "<nMeas>"

== system Grid_SensorLayout_SpatialAllignment_Clustering/OBJECT_TRACKER_SENSOR_FUSION/SENSOR_LAYOUT_AND_CHRACTERIZATION/SET_SENSOR_CALLIBRATION_PARAMETER/SET_CAMERA_SENSOR_PARAM/SET_CAMERA_INTRINSIC_PARAM/SET_CAMERA_INTRINSIC_PARAM ==
  SensorParam : Inport
  SensorID : Inport  Port=2
  Assignment : Assignment  DiagnosticForDimensions=Warning  IndexOptions=Index vector (port)  Indices=1  OutputSizes=1
  Bus Creator : BusCreator  Inputs=12  OutDataTypeStr=Bus: CameraIntrinsicParam  NonVirtualBus=on
  Bus Selector : BusSelector  OutputSignals=CameraType,RectificationMatrix,ProjectionMatrix,MaxRange,MaxAzimuth,MaxElevation,LongitudinalErrVariance,LateralErrVariance,ProbOfDetection,FalseAlarmRate,FOVRangePoints,FOVAzimuthPts
  Constant1 : Constant  Value=CAMERA_LONG_ERR_VAR
  Constant15 : Constant  Value=RADAR_PD
  Constant16 : Constant  Value=RADAR_FA
  Constant2 : Constant  Value=CAMERA_MAX_ELEVATION
  Constant3 : Constant  Value=CAMERA_LAT_ERR_VAR
  Constant4 : Constant  Value=CAMERA_MAX_RANGE
  Constant5 : Constant  Value=CAMERA_MAX_AZIMUTH
  Data Type Conversion : DataTypeConversion  OutDataTypeStr=uint8
  Selector{,1..3,5..6} (6 alike) : Selector  InputPortWidth=nCameraTypes  IndexOptions=Index vector (port)  Indices=[1 3]  OutputSizes=1
  Selector14 : Selector  InputPortWidth=nRadarTypes  IndexOptions=Index vector (port)  Indices=[1 3]  OutputSizes=1
  Selector15 : Selector  InputPortWidth=nRadarTypes  IndexOptions=Index vector (port)  Indices=[1 3]  OutputSizes=1
  Terminator{,1..7} (8 alike) : Terminator
  Out1 : Outport
  wires:
  Assignment/1 -> Out1/1
  SensorParam/1 -> [Param], Selector/1
  Selector/1 -> Bus Selector/1
  Bus Creator/1 -> Assignment/2
  SensorID/1 -> Selector/2, [SnsrTypeID]
  [Param] -> Assignment/1
  [SnsrTypeID] -> Assignment/3
  Constant5/1 -> Selector6/1
  Constant4/1 -> Selector5/1
  [SnsrTypeID] -> Selector15/2, Selector14/2, Selector3/2, Selector2/2, Selector1/2, Selector6/2, Selector5/2, Data Type Conversion/1
  Constant2/1 -> Selector1/1
  Constant15/1 -> Selector14/1
  Constant16/1 -> Selector15/1
  Bus Selector/1 -> Terminator/1  "<CameraType>"
  Bus Selector/2 -> Bus Creator/2  "<RectificationMatrix>"
  Bus Selector/4 -> Terminator3/1  "<MaxRange>"
  Bus Selector/3 -> Bus Creator/3  "<ProjectionMatrix>"
  Bus Selector/6 -> Terminator5/1  "<MaxElevation>"
  Bus Selector/7 -> Terminator6/1  "<LongitudinalErrVariance>"
  Bus Selector/8 -> Terminator7/1  "<LateralErrVariance>"
  Bus Selector/5 -> Terminator4/1  "<MaxAzimuth>"
  Selector5/1 -> Bus Creator/4  "MaxRange"
  Selector6/1 -> Bus Creator/5  "MaxAzimuth"
  Selector1/1 -> Bus Creator/6  "MaxElevation"
  Selector2/1 -> Bus Creator/7  "LongitudinalErrVariance"
  Selector3/1 -> Bus Creator/8  "LateralErrVariance"
  Constant1/1 -> Selector2/1
  Constant3/1 -> Selector3/1
  Selector14/1 -> Bus Creator/9  "ProbOfDetection"
  Selector15/1 -> Bus Creator/10  "FalseAlarmRate"
  Bus Selector/11 -> Bus Creator/11  "<FOVRangePoints>"
  Bus Selector/12 -> Bus Creator/12  "<FOVAzimuthPts>"
  Bus Selector/9 -> Terminator1/1  "<ProbOfDetection>"
  Bus Selector/10 -> Terminator2/1  "<FalseAlarmRate>"
  Data Type Conversion/1 -> Bus Creator/1  "CameraType"

== system Grid_SensorLayout_SpatialAllignment_Clustering/OBJECT_TRACKER_SENSOR_FUSION/SENSOR_LAYOUT_AND_CHRACTERIZATION/SET_SENSOR_CALLIBRATION_PARAMETER/SET_RADAR_SENSOR_PARAM/SET_RADAR_EXTRINSIC_PARAM/SET_RADAR_EXTRINSIC_PARAM ==
  SensorParam : Inport
  SensorID : Inport  Port=2
  Assignment : Assignment  DiagnosticForDimensions=Warning  IndexOptions=Index vector (port)  Indices=1  OutputSizes=1
  Bus Creator : BusCreator  Inputs=12  OutDataTypeStr=Bus: RadarExtrinsicParam  NonVirtualBus=on
  Bus Selector : BusSelector  OutputSignals=RadarID,RadarType,isActive,RotMat2D,TranslationVec,MountX,MountY,MountZ,MountYaw,MountPitch,MountRoll,nMeas
  CREATE_ROTATION_MATRIX_TRANSLATION_VECTOR : Subsystem
  Constant : Constant  Value=ACTIVATE_RAD
  Constant1 : Constant  Value=RAD_X_INSTALL
  Constant2 : Constant  Value=RAD_Y_INSTALL
  Constant3 : Constant  Value=RAD_YAW_INSTALL
  Constant4 : Constant  Value=RAD_nMeas
  Constant9 : Constant  Value=RAD_TYPE
  Data Type Conversion : DataTypeConversion  OutDataTypeStr=uint8
  Selector{,1..5,8} (7 alike) : Selector  InputPortWidth=nRadars  IndexOptions=Index vector (port)  Indices=[1 3]  OutputSizes=1
  Terminator{,1..8} (9 alike) : Terminator
  RadarSensorParam : Outport
  wires:
  Assignment/1 -> RadarSensorParam/1
  Constant/1 -> Selector1/1
  SensorParam/1 -> [Param], Selector/1
  Constant2/1 -> Selector3/1
  [SensorID] -> Selector5/2, Selector4/2, Selector3/2, Selector2/2, Selector1/2, Selector8/2, Data Type Conversion/1
  Constant3/1 -> Selector4/1
  Constant1/1 -> Selector2/1
  Selector/1 -> Bus Selector/1
  Bus Creator/1 -> Assignment/2
  Bus Selector/1 -> Terminator/1  "<RadarID>"
  SensorID/1 -> [SensorID], Selector/2
  [Param] -> Assignment/1
  [SensorID] -> Assignment/3
  Selector2/1 -> [MountX], Bus Creator/6  "MountX"
  Selector3/1 -> [MountY], Bus Creator/7  "MountY"
  [MountX] -> CREATE_ROTATION_MATRIX_TRANSLATION_VECTOR/2(xMount)
  [MountY] -> CREATE_ROTATION_MATRIX_TRANSLATION_VECTOR/3(yMount)
  Selector4/1 -> [MountYaw], Bus Creator/9  "MountYaw"
  [MountYaw] -> CREATE_ROTATION_MATRIX_TRANSLATION_VECTOR/1(yawInstall)
  CREATE_ROTATION_MATRIX_TRANSLATION_VECTOR/1(RotMatrx) -> [RotMat]
  CREATE_ROTATION_MATRIX_TRANSLATION_VECTOR/2(TranslationVector) -> [TransVec]
  Data Type Conversion/1 -> Bus Creator/1  "RadarID"
  Selector8/1 -> Bus Creator/2  "RadarType"
  Constant9/1 -> Selector8/1
  Selector1/1 -> Bus Creator/3  "isActive"
  [RotMat] -> Bus Creator/4  "RotMat2D"
  [TransVec] -> Bus Creator/5  "TranslationVec"
  Bus Selector/2 -> Terminator1/1  "<RadarType>"
  Bus Selector/3 -> Terminator2/1  "<isActive>"
  Bus Selector/4 -> Terminator3/1  "<RotMat2D>"
  Bus Selector/8 -> Bus Creator/8  "<MountZ>"
  Bus Selector/5 -> Terminator4/1  "<TranslationVec>"
  Bus Selector/7 -> Terminator6/1  "<MountY>"
  Bus Selector/6 -> Terminator5/1  "<MountX>"
  Bus Selector/9 -> Terminator8/1  "<MountYaw>"
  Bus Selector/11 -> Bus Creator/11  "<MountRoll>"
  Bus Selector/10 -> Bus Creator/10  "<MountPitch>"
  Selector5/1 -> Bus Creator/12  "nMeas"
  Constant4/1 -> Selector5/1
  Bus Selector/12 -> Terminator7/1  "<nMeas>"

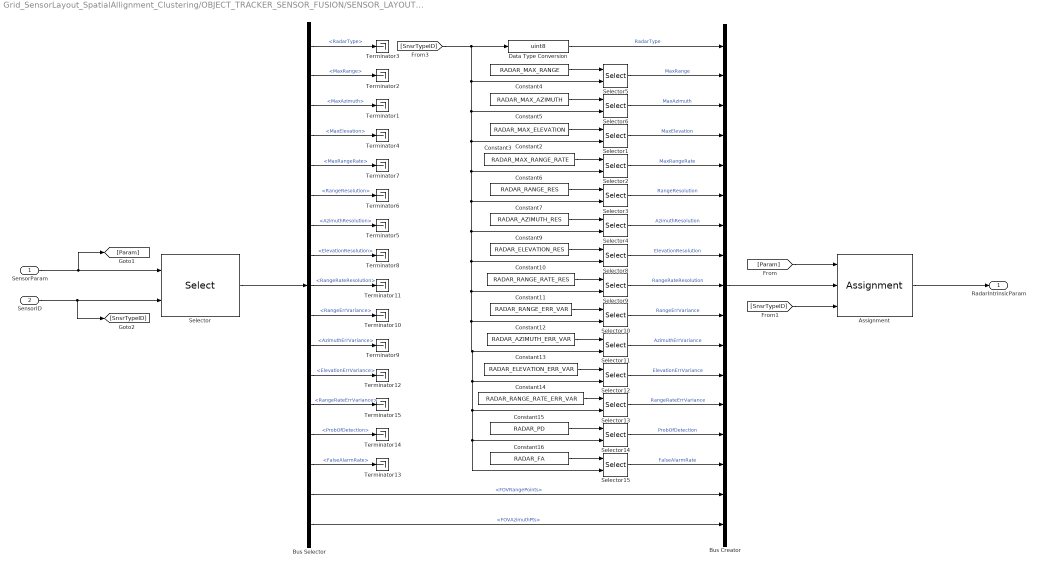
== system Grid_SensorLayout_SpatialAllignment_Clustering/OBJECT_TRACKER_SENSOR_FUSION/SENSOR_LAYOUT_AND_CHRACTERIZATION/SET_SENSOR_CALLIBRATION_PARAMETER/SET_RADAR_SENSOR_PARAM/SET_RADAR_INTRINSIC_PARAM/SET_RADAR_INTRINSIC_PARAM ==
  SensorParam : Inport
  SensorID : Inport  Port=2
  Assignment : Assignment  DiagnosticForDimensions=Warning  IndexOptions=Index vector (port)  Indices=1  OutputSizes=1
  Bus Creator : BusCreator  Inputs=17  OutDataTypeStr=Bus: RadarIntrinsicParam  NonVirtualBus=on
  Bus Selector : BusSelector  OutputSignals=RadarType,MaxRange,MaxAzimuth,MaxElevation,MaxRangeRate,RangeResolution,AzimuthResolution,ElevationResolution,RangeRateResolution,RangeErrVariance,AzimuthErrVariance,ElevationErrVariance,RangeRateErrVariance,ProbOfDetection,FalseAlarmRate,FOVRangePoints,FOVAzimuthPts
  Constant10 : Constant  Value=RADAR_RANGE_RATE_RES
  Constant11 : Constant  Value=RADAR_RANGE_ERR_VAR
  Constant12 : Constant  Value=RADAR_AZIMUTH_ERR_VAR
  Constant13 : Constant  Value=RADAR_ELEVATION_ERR_VAR
  Constant14 : Constant  Value=RADAR_RANGE_RATE_ERR_VAR
  Constant15 : Constant  Value=RADAR_PD
  Constant16 : Constant  Value=RADAR_FA
  Constant2 : Constant  Value=RADAR_MAX_ELEVATION
  Constant3 : Constant  Value=RADAR_MAX_RANGE_RATE
  Constant4 : Constant  Value=RADAR_MAX_RANGE
  Constant5 : Constant  Value=RADAR_MAX_AZIMUTH
  Constant6 : Constant  Value=RADAR_RANGE_RES
  Constant7 : Constant  Value=RADAR_AZIMUTH_RES
  Constant9 : Constant  Value=RADAR_ELEVATION_RES
  Data Type Conversion : DataTypeConversion  OutDataTypeStr=uint8
  Selector{,1..6,8..15} (15 alike) : Selector  InputPortWidth=nRadarTypes  IndexOptions=Index vector (port)  Indices=[1 3]  OutputSizes=1
  Terminator{1..15} (15 alike) : Terminator
  RadarIntrinsicParam : Outport
  wires:
  Assignment/1 -> RadarIntrinsicParam/1
  SensorParam/1 -> [Param], Selector/1
  Selector/1 -> Bus Selector/1
  Bus Creator/1 -> Assignment/2
  SensorID/1 -> [SnsrTypeID], Selector/2
  [Param] -> Assignment/1
  [SnsrTypeID] -> Assignment/3
  Bus Selector/17 -> Bus Creator/17  "<FOVAzimuthPts>"
  Bus Selector/16 -> Bus Creator/16  "<FOVRangePoints>"
  Constant5/1 -> Selector6/1
  Constant4/1 -> Selector5/1
  Bus Selector/3 -> Terminator1/1  "<MaxAzimuth>"
  Bus Selector/2 -> Terminator2/1  "<MaxRange>"
  Bus Selector/1 -> Terminator3/1  "<RadarType>"
  Selector6/1 -> Bus Creator/3  "MaxAzimuth"
  Selector5/1 -> Bus Creator/2  "MaxRange"
  [SnsrTypeID] -> Selector14/2, Selector15/2, Selector13/2, Selector12/2, Selector11/2, Selector10/2, Selector9/2, Selector8/2, Selector4/2, Selector3/2, Selector2/2, Selector1/2, Selector6/2, Selector5/2, Data Type Conversion/1
  Selector1/1 -> Bus Creator/4  "MaxElevation"
  Selector2/1 -> Bus Creator/5  "MaxRangeRate"
  Selector3/1 -> Bus Creator/6  "RangeResolution"
  Selector4/1 -> Bus Creator/7  "AzimuthResolution"
  Selector8/1 -> Bus Creator/8  "ElevationResolution"
  Constant2/1 -> Selector1/1
  Constant3/1 -> Selector2/1
  Constant6/1 -> Selector3/1
  Constant7/1 -> Selector4/1
  Constant9/1 -> Selector8/1
  Selector9/1 -> Bus Creator/9  "RangeRateResolution"
  Selector10/1 -> Bus Creator/10  "RangeErrVariance"
  Selector11/1 -> Bus Creator/11  "AzimuthErrVariance"
  Selector12/1 -> Bus Creator/12  "ElevationErrVariance"
  Selector13/1 -> Bus Creator/13  "RangeRateErrVariance"
  Selector14/1 -> Bus Creator/14  "ProbOfDetection"
  Selector15/1 -> Bus Creator/15  "FalseAlarmRate"
  Constant10/1 -> Selector9/1
  Constant11/1 -> Selector10/1
  Constant12/1 -> Selector11/1
  Constant13/1 -> Selector12/1
  Constant14/1 -> Selector13/1
  Constant15/1 -> Selector14/1
  Constant16/1 -> Selector15/1
  Bus Selector/4 -> Terminator4/1  "<MaxElevation>"
  Bus Selector/7 -> Terminator5/1  "<AzimuthResolution>"
  Bus Selector/6 -> Terminator6/1  "<RangeResolution>"
  Bus Selector/8 -> Terminator8/1  "<ElevationResolution>"
  Bus Selector/5 -> Terminator7/1  "<MaxRangeRate>"
  Bus Selector/11 -> Terminator9/1  "<AzimuthErrVariance>"
  Bus Selector/14 -> Terminator14/1  "<ProbOfDetection>"
  Bus Selector/10 -> Terminator10/1  "<RangeErrVariance>"
  Bus Selector/13 -> Terminator15/1  "<RangeRateErrVariance>"
  Bus Selector/12 -> Terminator12/1  "<ElevationErrVariance>"
  Bus Selector/15 -> Terminator13/1  "<FalseAlarmRate>"
  Bus Selector/9 -> Terminator11/1  "<RangeRateResolution>"
  Data Type Conversion/1 -> Bus Creator/1  "RadarType"

== system Grid_SensorLayout_SpatialAllignment_Clustering/OBJECT_TRACKER_SENSOR_FUSION/SIMPLIFIED_DBSCAN_FOR_RADAR_MEASUREMENT_GROUPING/DBSCAN_MEASUREMENT_GROUPING/FORM_CLUSTER/DBSCAN/DBSCAN_PROPAGATE_AND_EXPAND_CLUSTER ==
  nMeas : Inport
  measArray : Inport  Port=2
  CLSTR_DATA : Inport  Port=3
  CHECK_CONDITION : Subsystem
  DO_NOT_EXPAND_CLUSTER : Subsystem  TreatAsAtomicUnit=on
  EXPAND_CLUSTER : Subsystem  TreatAsAtomicUnit=on
  For Iterator : ForIterator  ResetStates=reset  IterationSource=external
  If : If  IfExpression=u1 == 0
  MERGE_SIGNALS : Subsystem
  CLSTR_DATA_UPD : Outport
  wires:
  nMeas/1 -> [nMeas], For Iterator/1
  For Iterator/1 -> CHECK_CONDITION/1(memberIdx)
  CLSTR_DATA/1 -> CHECK_CONDITION/2(CLSTR_DATA_INIT)
  CHECK_CONDITION/1(isMember) -> If/1
  MERGE_SIGNALS/1(CLSTR_DATA) -> CHECK_CONDITION/3(CLSTR_DATA_PREV), CLSTR_DATA_UPD/1
  If/1 -> DO_NOT_EXPAND_CLUSTER/Action
  If/2 -> EXPAND_CLUSTER/Action
  CHECK_CONDITION/2(MeasIndex) -> [x_i]
  DO_NOT_EXPAND_CLUSTER/1(CLSTR_DATA_NO_UPD) -> MERGE_SIGNALS/1(CLSTR_NO_UPD)
  CHECK_CONDITION/3(CLSTR_DATA) -> DO_NOT_EXPAND_CLUSTER/1(CLSTR_DATA), EXPAND_CLUSTER/1(CLSTR_DATA)
  [nMeas] -> EXPAND_CLUSTER/2(nMeas)
  [x_i] -> EXPAND_CLUSTER/3(idx_i)
  measArray/1 -> EXPAND_CLUSTER/4(measArray)
  EXPAND_CLUSTER/1(CLSTR_DATA_UPD) -> MERGE_SIGNALS/2(CLSTR_UPD)

== system Grid_SensorLayout_SpatialAllignment_Clustering/OBJECT_TRACKER_SENSOR_FUSION/SIMPLIFIED_DBSCAN_FOR_RADAR_MEASUREMENT_GROUPING/DBSCAN_MEASUREMENT_GROUPING/FORM_CLUSTER/DBSCAN/INITIALIZE_CLUSTER ==
  CLUSTERING_DATA : Inport
  RAD_MEAS_CTS : Inport  Port=2
  idx_i : Inport  Port=3
  Add2 : Sum
  Assignment1 : Assignment  NumberOfDimensions=2  DiagnosticForDimensions=Warning  IndexOptions=Assign all,Index vector (dialog)  Indices=1,1  OutputSizes=1,1
  Bus Creator : BusCreator  Inputs=7  OutDataTypeStr=Bus: CLUSTER_DATA_STRUCT_SNSR  NonVirtualBus=on
      settings: InheritFromInputs=off
  Bus Selector : BusSelector  OutputSignals=nClusters,ClusterMember
  Bus Selector1 : BusSelector  OutputSignals=ValidCumulativeMeasCount
  Bus Selector2 : BusSelector  OutputSignals=ClusterCenter,ClusterCovariance,ClusterSizes,ClusterToMeasAssignment,isMeasVisitedFlag,nClusters,ClusterMember
  Constant3 : Constant  Value=uint16(1)
  Data Type Conversion : DataTypeConversion  OutDataTypeStr=uint16
  Data Type Conversion1 : DataTypeConversion  OutDataTypeStr=uint16
  Selector : Selector  NumberOfDimensions=2  InputPortWidth=3  IndexOptions=Select all,Index vector (port)  Indices=[1 3],1  OutputSizes=1,1
  Terminator1 : Terminator
  Terminator2 : Terminator
  Width : Width
  nRadMeas : Outport
  CLUSTER_DATA : Outport  Port=2
  wires:
  CLUSTERING_DATA/1 -> Bus Selector2/1, Bus Selector/1
  Bus Selector/1 -> Add2/1  "<nClusters>"
  RAD_MEAS_CTS/1 -> Bus Selector1/1
  Add2/1 -> Data Type Conversion/1
  Constant3/1 -> Add2/2
  Data Type Conversion/1 -> [B]
  Bus Selector2/1 -> Bus Creator/1  "<ClusterCenter>"
  Bus Selector2/2 -> Bus Creator/2  "<ClusterCovariance>"
  Bus Selector2/3 -> Bus Creator/3  "<ClusterSizes>"
  Bus Selector2/4 -> Bus Creator/4  "<ClusterToMeasAssignment>"
  Bus Selector2/5 -> Bus Creator/5  "<isMeasVisitedFlag>"
  Bus Selector2/6 -> Terminator1/1  "<nClusters>"
  [B] -> Bus Creator/6  "nClusters"
  Bus Creator/1 -> CLUSTER_DATA/1
  Bus Selector/2 -> Assignment1/1  "<ClusterMember>"
  Assignment1/1 -> [C]
  idx_i/1 -> Data Type Conversion1/1
  [C] -> Bus Creator/7  "ClusterMember"
  Bus Selector2/7 -> Terminator2/1  "<ClusterMember>"
  Data Type Conversion1/1 -> Assignment1/2
  Selector/1 -> nRadMeas/1
  Width/1 -> Selector/2
  Bus Selector1/1 -> Width/1, Selector/1  "<ValidCumulativeMeasCount>"

== system Grid_SensorLayout_SpatialAllignment_Clustering/OBJECT_TRACKER_SENSOR_FUSION/SIMPLIFIED_DBSCAN_FOR_RADAR_MEASUREMENT_GROUPING/DBSCAN_MEASUREMENT_GROUPING/FORM_CLUSTER/DBSCAN/Subsystem ==
  CLSTR_DATA : Inport
  Bus Selector : BusSelector  OutputSignals=ClusterSizes,nClusters
  Selector : Selector  NumberOfDimensions=2  InputPortWidth=3  IndexOptions=Select all,Index vector (port)  Indices=[1 3],1  OutputSizes=1,1
  ClstrSize : Outport
  wires:
  Bus Selector/2 -> Selector/2  "<nClusters>"
  Bus Selector/1 -> Selector/1  "<ClusterSizes>"
  CLSTR_DATA/1 -> Bus Selector/1
  Selector/1 -> ClstrSize/1

== system Grid_SensorLayout_SpatialAllignment_Clustering/OBJECT_TRACKER_SENSOR_FUSION/SPATIAL_ALLIGNMENT/CAMERA_MEASUREMENTS_SPATIAL_ALLIGNMENT/For Iterator Subsystem/For Iterator Subsystem/CoordinateTransformation1 ==
  meas : Inport
  SensorParam : Inport  Port=2
  Action Port : ActionPort  ActionType=then
  InfoExtractor : Subsystem
  Meas_Noise_Cov_Transformation : Subsystem
  Position_Transformation : Subsystem
  Subsystem : Subsystem
  Velocity_Transformation : Subsystem
  measUpd : Outport
  wires:
  meas/1 -> InfoExtractor/1(In1)
  SensorParam/1 -> InfoExtractor/2(In2)
  Velocity_Transformation/1(VelXcts) -> [VxCTS]  "vxCTS"
  InfoExtractor/5(RotMat2D) -> Velocity_Transformation/3(RotMatrix2D), Meas_Noise_Cov_Transformation/1(RotMatrix), [RotMat]
  InfoExtractor/4(<vy>) -> Velocity_Transformation/2(Vy)
  InfoExtractor/3(<vx>) -> Velocity_Transformation/1(Vx)
  InfoExtractor/1(<px>) -> Position_Transformation/1(Px)
  InfoExtractor/2(<py>) -> Position_Transformation/2(Py)
  InfoExtractor/7(MeasNoiseCov) -> Meas_Noise_Cov_Transformation/2(MeasCovarience)
  [RotMat] -> Position_Transformation/3(RotationMat)
  [TransVector] -> Position_Transformation/4(TranslationVector)
  InfoExtractor/6(TransVec2D) -> [TransVector]
  Position_Transformation/1(PosXcts) -> Subsystem/1(pxCTS)
  Meas_Noise_Cov_Transformation/1(MeasCovTransformed) -> Subsystem/5(covCTS)
  Position_Transformation/2(PosYcts) -> Subsystem/2(pyCTS)
  Velocity_Transformation/2(VelYcts) -> [VyCTS]  "vyCTS"
  [VxCTS] -> Subsystem/3(vxCTS)
  [VyCTS] -> Subsystem/4(vyCTS)
  Subsystem/1(measUpd) -> measUpd/1
